simulink model "nonlinear_truck"  (R2017b)
settings: Solver=VariableStepAuto  StartTime=0.0  StopTime=50.0  RelTol=1e-3
values from neighbouring files (symbols this model uses):
  init_conditions_high = [start_x start_y zeros(1, n_h2h) start_angle zeros(1, n_r2r) zeros(1, n_r2h) 0]    [handle_data.m]
  init_conditions_low = [start_x start_y zeros(1, n_h2h) start_angle zeros(1, n_r2r)]    [handle_data.m]
  Ts = mean(diff(in.Time))    [handle_data.m]    (also in hastighet2hastighet.m = 0.025; rotationshastighet2hastighet.m = 0.025; rotationshastighet2rotationshastighet.m = 0.025)
settings Model: Creator=danie  LastModifiedBy=danie

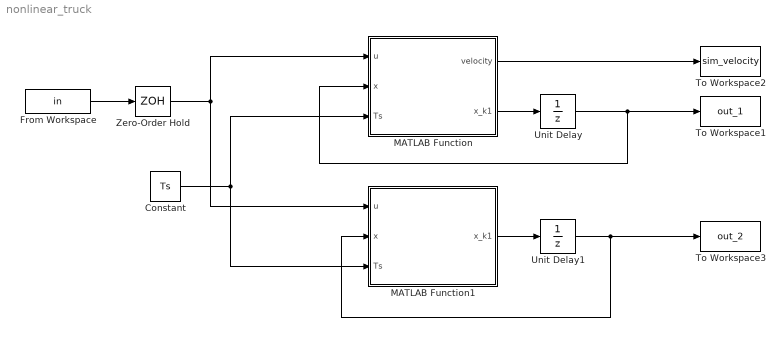
== system nonlinear_truck ==
  Constant : Constant  Value=Ts
  From Workspace : FromWorkspace  VariableName=in  SampleTime=Ts  OutputAfterFinalValue=Setting to zero
  MATLAB Function : MATLAB Function  TreatAsAtomicUnit=on
  MATLAB Function1 : MATLAB Function  TreatAsAtomicUnit=on
  To Workspace1 : ToWorkspace  VariableName=out_1  SaveFormat=Timeseries  SampleTime=-1
  To Workspace2 : ToWorkspace  VariableName=sim_velocity  SaveFormat=Timeseries  SampleTime=-1
  To Workspace3 : ToWorkspace  VariableName=out_2  SaveFormat=Timeseries  SampleTime=-1
  Unit Delay : UnitDelay  InitialCondition=init_conditions_high  SampleTime=Ts
  Unit Delay1 : UnitDelay  InitialCondition=init_conditions_low  SampleTime=Ts
  Zero-Order Hold : ZeroOrderHold  SampleTime=Ts
  wires:
  MATLAB Function/2(x_k1) -> Unit Delay/1
  MATLAB Function/1(velocity) -> To Workspace2/1
  Unit Delay/1 -> To Workspace1/1, MATLAB Function/2(x)
  From Workspace/1 -> Zero-Order Hold/1
  Zero-Order Hold/1 -> MATLAB Function/1(u), MATLAB Function1/1(u)
  Constant/1 -> MATLAB Function1/3(Ts), MATLAB Function/3(Ts)
  Unit Delay1/1 -> MATLAB Function1/2(x), To Workspace3/1
  MATLAB Function1/1(x_k1) -> Unit Delay1/1

== matlab function nonlinear_truck/MATLAB Function1 ==
  data: u input; x_k1 output; x input; Ts input
function x_k1  = discrete_truck_2(u, x, Ts)
% Olinjär model av trucken. Tar en hastighet och vinkelhastighet som
% insignal. Ger position som utsignal.

% h2h = "Linjär hastighet till linjär hastighet"
% r2r = "Rotationshastighet till rotationshastighet"
% r2h = "Rotationshastighet till linjär hastighet"
% Dessa beskriver överföringen från de önskade insignalerna till de
% hastigheter som trucken faktiskt kör med.


% Tillstånd

% x1 =          truckens x-koordinat i världskoordinatsystemet
% x2 =          truckens y-koordinat i världskoordinatsystemet

% x3-xN =       interna tillstånd som beskriver överföringen från inskickad
%               hastighet till den hastighet som fås i verkligheten. 
%               N = 3 + antal tillstånd i h2h - 1

% x(N+1) =      truckens rotation i förhållande till sin omgivning

% x(N+2)-x(M) = interna tillstånd som beskriver överföringen från inskickad
%               rotationshastighet till den rotationshastighet som fås i verkligheten.
%               M = N + 2 + antal tillstånd i r2r - 1;

% x(M+1) =      Beskriver hur truckens hastighet påverkas av
%               rotationshastighet.


% Ladda in linjära överföringsmatriser som tagits fram tidigare.
h2h = load('h2h_low');
r2r = load('r2r_low');
n_h2h = size(h2h.Ah2h, 1);
n_r2r = size(r2r.Ar2r, 1);


x_k1 = zeros(3+n_h2h+n_r2r,1);

% Parametrar för finanpassning
scale_v = 0.9;
scale_r = 0.7;

% Beräkna hastigheten.
orig_vel = h2h.Ch2h * x(3:3+n_h2h-1) + h2h.Dh2h * u(1);
velocity = scale_v*orig_vel;
   
% Position
x_k1(1) = x(1) + velocity * cos( x(3+n_h2h) )*Ts;
x_k1(2) = x(2) + velocity * sin( x(3+n_h2h) )*Ts;

% Överföring hastighet till hastighet
x_k1(3:3+n_h2h-1) = h2h.Ah2h * x(3:3+n_h2h-1) + h2h.Bh2h * u(1);

% Rotation
x_k1(3+n_h2h) = x(3+n_h2h) + scale_r*(r2r.Cr2r * x(4+n_h2h:4+n_h2h+n_r2r-1) + r2r.Dr2r * u(2)) *Ts;

% Överföring rotationshastighet till rotationshastighet
x_k1(4+n_h2h:4+n_h2h+n_r2r-1) = r2r.Ar2r * x(4+n_h2h:4+n_h2h+n_r2r-1) + r2r.Br2r * u(2);


end

== matlab function nonlinear_truck/MATLAB Function ==
  data: velocity output; u input; x_k1 output; x input; Ts input
function [velocity,x_k1] = discrete_truck_1(u, x, Ts)
% Olinjär model av trucken. Tar en hastighet och vinkelhastighet som
% insignal. Ger position som utsignal.

% h2h = "Linjär hastighet till linjär hastighet"
% r2r = "Rotationshastighet till rotationshastighet"
% r2h = "Rotationshastighet till linjär hastighet"
% Dessa beskriver överföringen från de önskade insignalerna till de
% hastigheter som trucken faktiskt kör med.


% Tillstånd

% x1 =          truckens x-koordinat i världskoordinatsystemet
% x2 =          truckens y-koordinat i världskoordinatsystemet

% x3-xN =       interna tillstånd som beskriver överföringen från inskickad
%               hastighet till den hastighet som fås i verkligheten. 
%               N = 3 + antal tillstånd i h2h - 1

% x(N+1) =      truckens rotation i förhållande till sin omgivning

% x(N+2)-x(M) = interna tillstånd som beskriver överföringen från inskickad
%               rotationshastighet till den rotationshastighet som fås i verkligheten.
%               M = N + 2 + antal tillstånd i r2r - 1;

% x(M+1) =      Beskriver hur truckens hastighet påverkas av
%               rotationshastighet.


% Ladda in linjära överföringsmatriser som tagits fram tidigare.
h2h = load('h2h_high');
r2r = load('r2r_high');
r2h = load('r2h');
n_r2h = size(r2h.Ar2h, 1);
n_h2h = size(h2h.Ah2h, 1);
n_r2r = size(r2r.Ar2r, 1);

x_k1 = zeros(4+n_h2h+n_r2r+n_r2h,1);

% Parametrar för finanpassning
scale_v = 0.9;
scale_r = 0.75;
scale_r2h = 0.01;


% Beräkna hastigheten. Modellen av högre ordning tar hänsyn till
% rotationshastighetens påverkan på den linjära hastigheten.
orig_vel = h2h.Ch2h * x(3:3+n_h2h-1) + h2h.Dh2h * u(1);
velocity = scale_v*orig_vel - scale_r2h*sign(orig_vel) * r2h.Cr2h * x(4+n_h2h+n_r2r:4+n_h2h+n_r2r+n_r2h-1);
  
% Position
x_k1(1) = x(1) + velocity * cos( x(3+n_h2h) )*Ts;
x_k1(2) = x(2) + velocity * sin( x(3+n_h2h) )*Ts;

% Överföring hastighet till hastighet
x_k1(3:3+n_h2h-1) = h2h.Ah2h * x(3:3+n_h2h-1) + h2h.Bh2h * u(1);

% Rotation
x_k1(3+n_h2h) = x(3+n_h2h) + scale_r*(r2r.Cr2r * x(4+n_h2h:4+n_h2h+n_r2r-1) + r2r.Dr2r * u(2)) *Ts;

% Överföring vinkelhastighet till vinkelhastighet
x_k1(4+n_h2h:4+n_h2h+n_r2r-1) = r2r.Ar2r * x(4+n_h2h:4+n_h2h+n_r2r-1) + r2r.Br2r * u(2);

% Överföring rotationshastighet till hastighet
x_k1(4+n_h2h+n_r2r:4+n_h2h+n_r2r+n_r2h-1) = r2h.Ar2h*x(4+n_h2h+n_r2r:4+n_h2h+n_r2r+n_r2h-1) + ...
                                            r2h.Br2h * abs( ( u(2)-x(4+n_h2h+n_r2r+n_r2h) ) / Ts);

x_k1(4+n_h2h+n_r2r+n_r2h) = u(2);


end
